simulink model "LQR_Rocket"  (R2020a)
settings: Solver=VariableStepAuto  StartTime=0.0  StopTime=4000  RelTol=1e-3
values from neighbouring files (symbols this model uses):
  A = [0 1 0 0    0                  0 ... (first row only)    [rocket_ABCD.m]
  B = [0              0        0 ... (first row only)    [rocket_ABCD.m]
  C = [1 0 0 0 0 0 ... (first row only)    [rocket_ABCD.m]
  x0 = Simulink.BlockDiagram.getInitialState('LQGrocket')    [rocket_main_LQG.m]    (also in rocket_main_LQR.m = [10 0 1000 0 deg2rad(-10) 0]')
undefined symbols (not defined in the file or in its folder): K
libraries: simulink_extras x1
settings Model: Creator=Aashkaran Dhillon  LastModifiedBy=Aashkaran Dhillon

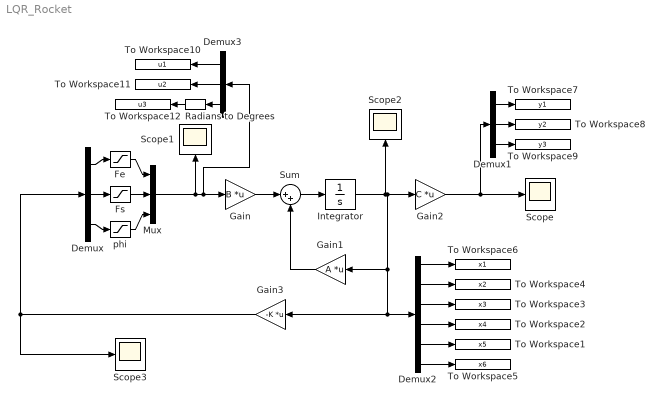
== system LQR_Rocket ==
  Demux : Demux  Outputs=3
  Demux1 : Demux  Outputs=3
  Demux2 : Demux  Outputs=6
  Demux3 : Demux  Outputs=3
  Fe : Saturate  UpperLimit=0  LowerLimit=-845e3  LinearizeAsGain=off
  Fs : Saturate  UpperLimit=130  LowerLimit=-130  LinearizeAsGain=off
  Gain : Gain  Gain=B  Multiplication=Matrix(K*u)
  Gain1 : Gain  Gain=A  Multiplication=Matrix(K*u)
  Gain2 : Gain  Gain=C  Multiplication=Matrix(K*u)
  Gain3 : Gain  Gain=-K  Multiplication=Matrix(K*u)
  Integrator : Integrator  InitialCondition=x0
  Mux : Mux  Inputs=3
  Radians to Degrees : simulink_extras/Transformations/Radians to Degrees
  Scope{,1..3} (4 alike) : Scope
  Sum : Sum  Inputs=|++
  To Workspace1 : ToWorkspace  VariableName=x5  SaveFormat=Timeseries  SampleTime=-1
  To Workspace10 : ToWorkspace  VariableName=u1  SaveFormat=Timeseries  SampleTime=-1
  To Workspace11 : ToWorkspace  VariableName=u2  SaveFormat=Timeseries  SampleTime=-1
  To Workspace12 : ToWorkspace  VariableName=u3  SaveFormat=Timeseries  SampleTime=-1
  To Workspace2 : ToWorkspace  VariableName=x4  SaveFormat=Timeseries  SampleTime=-1
  To Workspace3 : ToWorkspace  VariableName=x3  SaveFormat=Timeseries  SampleTime=-1
  To Workspace4 : ToWorkspace  VariableName=x2  SaveFormat=Timeseries  SampleTime=-1
  To Workspace5 : ToWorkspace  VariableName=x6  SaveFormat=Timeseries  SampleTime=-1
  To Workspace6 : ToWorkspace  VariableName=x1  SaveFormat=Timeseries  SampleTime=-1
  To Workspace7 : ToWorkspace  VariableName=y1  SaveFormat=Timeseries  SampleTime=-1
  To Workspace8 : ToWorkspace  VariableName=y2  SaveFormat=Timeseries  SampleTime=-1
  To Workspace9 : ToWorkspace  VariableName=y3  SaveFormat=Timeseries  SampleTime=-1
  phi : Saturate  UpperLimit=deg2rad(15)  LowerLimit=deg2rad(-15)  LinearizeAsGain=off
  wires:
  Integrator/1 -> Gain2/1, Gain1/1, Demux2/1, Gain3/1, Scope2/1
  Gain2/1 -> Demux1/1, Scope/1
  Sum/1 -> Integrator/1
  Gain/1 -> Sum/1
  Gain1/1 -> Sum/2
  Demux2/6 -> To Workspace5/1
  Demux2/1 -> To Workspace6/1
  Demux2/2 -> To Workspace4/1
  Demux2/4 -> To Workspace2/1
  Demux2/3 -> To Workspace3/1
  Demux2/5 -> To Workspace1/1
  Demux1/1 -> To Workspace7/1
  Demux1/3 -> To Workspace9/1
  Demux1/2 -> To Workspace8/1
  Demux3/2 -> To Workspace11/1
  Demux3/1 -> To Workspace10/1
  Demux3/3 -> Radians to Degrees/1
  Radians to Degrees/1 -> To Workspace12/1
  Gain3/1 -> Demux/1, Scope3/1
  Fe/1 -> Mux/1
  Demux/1 -> Fe/1
  Demux/3 -> phi/1
  phi/1 -> Mux/3
  Demux/2 -> Fs/1
  Fs/1 -> Mux/2
  Mux/1 -> Scope1/1, Demux3/1, Gain/1
